simulink model "sesion1C_indentplanta"  (R2020b)
settings: Solver=VariableStepAuto  StartTime=0.0  StopTime=10.0  RelTol=1e-3
settings Model: Creator=Catolica  LastModifiedBy=Catolica

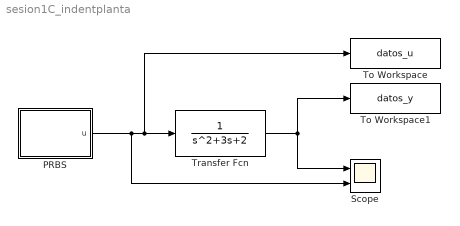
== system sesion1C_indentplanta ==
  PRBS : MATLAB Function  TreatAsAtomicUnit=on  SystemSampleTime=0.04
  Scope : Scope  NumInputPorts=2
  To Workspace : ToWorkspace  VariableName=datos_u  SampleTime=0.04
  To Workspace1 : ToWorkspace  VariableName=datos_y  SampleTime=0.04
  Transfer Fcn : TransferFcn  Denominator="[1 3  2]"
  wires:
  PRBS/1(u) -> Scope/2, To Workspace/1, Transfer Fcn/1
  Transfer Fcn/1 -> To Workspace1/1, Scope/1

== matlab function sesion1C_indentplanta/PRBS ==
  data: u output
function u = fcn()
persistent b1
persistent b2
persistent b3
persistent b4
persistent b5
persistent b6
persistent b7
if isempty(b1),
    b1=1;
    b2=0;
    b3=0;
    b4=0;
    b5=1;
    b6=1;
    b7=1;
end;
a3=1; a7=1;

b=mod(a3*b3+a7*b7,2);
if b==0,
    u=0
else
    u=1
end;
b7=b6;
b6=b5;
b5=b4;
b4=b3;
b3=b2;
b2=b1;
b1=b;
